simulink model "ArmModSegSep"  (R2017a)
settings: Solver=VariableStepAuto  StartTime=0.0  StopTime=length(gyroyaccel(:,1))/100  RelTol=1e-3
undefined symbols (not defined in the file): sigbuilder_block
libraries: vrlib x8, sharedtransform x6
settings Model: Creator=erich  LastModifiedBy=MarioAndres

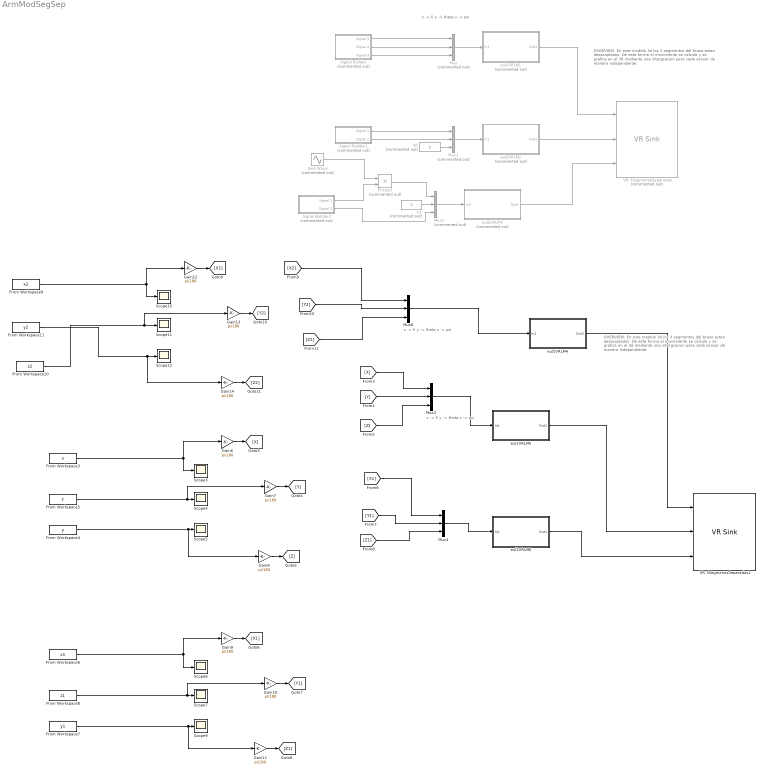
== system ArmModSegSep ==
  note: OVERVIEW:
      | En este modelo 3d los 3 segmentos del
      | brazo estan desacoplados. De esta forma
      | el movimiento se calcula y se grafica en el
      | 3d mediante una intergracion para cada
      | sensor de manera independiente.
  note: x -> fi
      | y -> theta
      | z -> psi
  note: OVERVIEW:
      | En este modelo 3d los 3 segmentos del
      | brazo estan desacoplados. De esta forma
      | el movimiento se calcula y se grafica en el
      | 3d mediante una intergracion para cada
      | sensor de manera independiente.
  note: x -> fi
      | y -> theta
      | z -> psi
  note: x -> fi
      | y -> theta
      | z -> psi
  From Workspace10 : FromWorkspace  VariableName=z2  SampleTime=0.01
  From Workspace11 : FromWorkspace  VariableName=y2  SampleTime=0.01
  From Workspace3 : FromWorkspace  VariableName=x  SampleTime=0.01
  From Workspace4 : FromWorkspace  VariableName=y  SampleTime=0.01
  From Workspace5 : FromWorkspace  VariableName=z  SampleTime=0.01
  From Workspace6 : FromWorkspace  VariableName=x1  SampleTime=0.01
  From Workspace7 : FromWorkspace  VariableName=y1  SampleTime=0.01
  From Workspace8 : FromWorkspace  VariableName=z1  SampleTime=0.01
  From Workspace9 : FromWorkspace  VariableName=x2  SampleTime=0.01
  Gain{6..14} (9 alike) : Gain  Gain=pi/180
  Mux : Mux  Commented=on  Inputs=3
  Mux1 : Mux  Commented=on  Inputs=3
  Mux2 : Mux  Commented=on  Inputs=3
  Mux3 : Mux  Inputs=3
  Mux4 : Mux  Inputs=3
  Mux6 : Mux  Inputs=3
  Product : Product  Commented=on
  Scope{3..7,9..12} (9 alike) : Scope
  Signal Builder : Subsystem  Tag=STV Subsys  Commented=on  LoadFcn=sigbuilder_block('load');  StartFcn=sigbuilder_block('start');  StopFcn=sigbuilder_block('stop');  ClipboardFcn=sigbuilder_block('clipboard');  mask(Sigbuilder block){tuvar=[0:10]}
      mask help: Simulink:masks:SigbuilderBlock_MD
      mask init:
      | if ~strcmp(get_param(bdroot(gcbh),'SimulationStatus'),'stopped') tuvar = sigbuilder_block('maskInit'); end
      settings: CopyFcn=sigbuilder_block('copy');  DeleteFcn=sigbuilder_block('delete');  ModelCloseFcn=sigbuilder_block('modelClose');  PreSaveFcn=sigbuilder_block('preSave');  PauseFcn=sigbuilder_block('pause');  ContinueFcn=sigbuilder_block('continue');  NameChangeFcn=sigbuilder_block('namechange');  OpenFcn=sigbuilder_block('open',[204 106.5 550.5 359.25 ]);  CloseFcn=sigbuilder_block('close');
      mask Display: plot(0, 0, 100, 100,[2, 2, 32, 32, 2], [68, 8, 8, 68, 68],[32, 2], [38, 38], [32, 19, 2],[53, 60, 44], [32, 17, 17, 2],[16, 16, 31, 31]);txt = getActiveGroup(gcbh);text(2, 100, txt,'verticalAlignment', 'top');
  Signal Builder1 : Subsystem  Tag=STV Subsys  Commented=on  LoadFcn=sigbuilder_block('load');  StartFcn=sigbuilder_block('start');  StopFcn=sigbuilder_block('stop');  ClipboardFcn=sigbuilder_block('clipboard');  mask(Sigbuilder block){tuvar=[0:10]}
      mask help: Simulink:masks:SigbuilderBlock_MD
      mask init:
      | if ~strcmp(get_param(bdroot(gcbh),'SimulationStatus'),'stopped') tuvar = sigbuilder_block('maskInit'); end
      settings: CopyFcn=sigbuilder_block('copy');  DeleteFcn=sigbuilder_block('delete');  ModelCloseFcn=sigbuilder_block('modelClose');  PreSaveFcn=sigbuilder_block('preSave');  PauseFcn=sigbuilder_block('pause');  ContinueFcn=sigbuilder_block('continue');  NameChangeFcn=sigbuilder_block('namechange');  OpenFcn=sigbuilder_block('open',[437.25 153 550.5 359.25 ]);  CloseFcn=sigbuilder_block('close');
      mask Display: plot(0, 0, 100, 100,[2, 2, 32, 32, 2], [68, 8, 8, 68, 68],[32, 2], [38, 38], [32, 19, 2],[53, 60, 44], [32, 17, 17, 2],[16, 16, 31, 31]);txt = getActiveGroup(gcbh);text(2, 100, txt,'verticalAlignment', 'top');
  Signal Builder2 : Subsystem  Tag=STV Subsys  Commented=on  LoadFcn=sigbuilder_block('load');  StartFcn=sigbuilder_block('start');  StopFcn=sigbuilder_block('stop');  ClipboardFcn=sigbuilder_block('clipboard');  mask(Sigbuilder block){tuvar=[0:10]}
      mask help: Simulink:masks:SigbuilderBlock_MD
      mask init:
      | if ~strcmp(get_param(bdroot(gcbh),'SimulationStatus'),'stopped') tuvar = sigbuilder_block('maskInit'); end
      settings: CopyFcn=sigbuilder_block('copy');  DeleteFcn=sigbuilder_block('delete');  ModelCloseFcn=sigbuilder_block('modelClose');  PreSaveFcn=sigbuilder_block('preSave');  PauseFcn=sigbuilder_block('pause');  ContinueFcn=sigbuilder_block('continue');  NameChangeFcn=sigbuilder_block('namechange');  OpenFcn=sigbuilder_block('open',[437.25 153 550.5 359.25 ]);  CloseFcn=sigbuilder_block('close');
      mask Display: plot(0, 0, 100, 100,[2, 2, 32, 32, 2], [68, 8, 8, 68, 68],[32, 2], [38, 38], [32, 19, 2],[53, 60, 44], [32, 17, 17, 2],[16, 16, 31, 31]);txt = getActiveGroup(gcbh);text(2, 100, txt,'verticalAlignment', 'top');
  Sine Wave : Sin  Commented=on  Amplitude=pi/10  Frequency=3  SampleTime=0
  VR 3SegmenosSeparados : vrlib/VR Sink  Commented=on  InstantiateOnLoad=on  SampleTime=0.1  ViewEnable=on  RemoteChange=off  RemoteView=off  FieldsWritten=Sphere_HombroCodo.rotation.4.1.1.double#Sphere_CodoMano.rotation.4.1.1.double#Sphere_Mano.rotation.4.1.1.double  WorldFileName=VM\VM_HCM_separados.wrl  AutoView=off  VideoDimensions=[]  AllowVariableSize=off
      settings: SourceProductBaseCode=VR
  VR 3SegmenosSeparados1 : vrlib/VR Sink  InstantiateOnLoad=on  SampleTime=0.01  ViewEnable=on  RemoteChange=off  RemoteView=off  FieldsWritten=Sphere_HombroCodo.rotation.4.1.1.double#Sphere_CodoMano.rotation.4.1.1.double#Sphere_Mano.rotation.4.1.1.double  WorldFileName=VM\VM_HCM_separados.wrl  AutoView=off  VideoDimensions=[]  AllowVariableSize=off
      settings: SourceProductBaseCode=VR
  eul2VRLM1 : Subsystem  Commented=on
  eul2VRLM2 : Subsystem  Commented=on
  eul2VRLM3 : Subsystem  Commented=on
  eul2VRLM4 : Subsystem
  eul2VRLM5 : Subsystem
  eul2VRLM6 : Subsystem
  k0 : Constant  Commented=on  Value=0
  k1 : Constant  Commented=on  Value=0
  wires:
  Signal Builder2/1(Signal 1) -> Product/2
  k1/1 -> Mux2/2
  Signal Builder2/2(Signal 2) -> Mux2/3
  Sine Wave/1 -> Product/1
  Signal Builder1/2(Signal 2) -> Mux1/2
  Product/1 -> Mux2/1
  Mux/1 -> eul2VRLM1/1(In1)
  Signal Builder1/1(Signal 1) -> Mux1/1
  Mux2/1 -> eul2VRLM3/1(In1)
  Mux1/1 -> eul2VRLM2/1(In1)
  k0/1 -> Mux1/3
  Signal Builder/2(Signal 2) -> Mux/2
  Signal Builder/3(Signal 3) -> Mux/3
  Signal Builder/1(Signal 1) -> Mux/1
  eul2VRLM1/1(Out1) -> VR 3SegmenosSeparados/1
  eul2VRLM2/1(Out1) -> VR 3SegmenosSeparados/2
  eul2VRLM3/1(Out1) -> VR 3SegmenosSeparados/3
  Mux6/1 -> eul2VRLM4/1(In1)
  From Workspace6/1 -> Gain9/1, Scope6/1
  [X2] -> Mux6/1
  Gain12/1 -> [X2]
  Gain11/1 -> [Z1]
  From Workspace8/1 -> Gain10/1, Scope7/1
  Gain14/1 -> [Z2]
  [X1] -> Mux4/1
  Gain13/1 -> [Y2]
  Gain7/1 -> [Y]
  [X] -> Mux3/1
  From Workspace9/1 -> Gain12/1, Scope10/1
  Gain10/1 -> [Y1]
  From Workspace5/1 -> Gain7/1, Scope4/1
  [Z2] -> Mux6/3
  eul2VRLM5/1(Out1) -> VR 3SegmenosSeparados1/2
  [Y1] -> Mux4/2
  [Z] -> Mux3/3
  eul2VRLM6/1(Out1) -> VR 3SegmenosSeparados1/3
  From Workspace3/1 -> Scope3/1, Gain6/1
  [Y] -> Mux3/2
  From Workspace7/1 -> Gain11/1, Scope9/1
  Gain9/1 -> [X1]
  eul2VRLM4/1(Out1) -> VR 3SegmenosSeparados1/1
  Gain6/1 -> [X]
  Gain8/1 -> [Z]
  [Y2] -> Mux6/2
  From Workspace4/1 -> Gain8/1, Scope5/1
  [Z1] -> Mux4/3
  Mux3/1 -> eul2VRLM5/1(In1)
  Mux4/1 -> eul2VRLM6/1(In1)
  From Workspace11/1 -> Gain14/1, Scope12/1
  From Workspace10/1 -> Gain13/1, Scope11/1

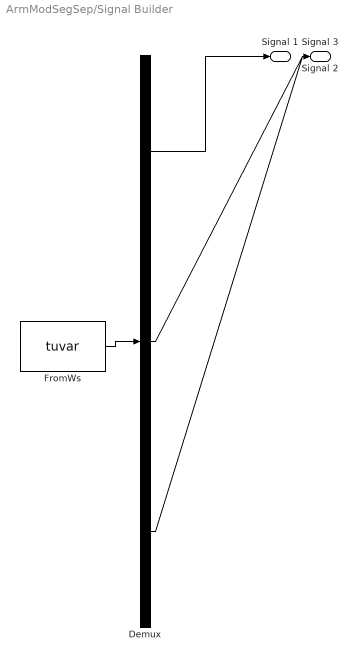
== system ArmModSegSep/Signal Builder ==
  Demux : Demux  Tag=STV Demux  Outputs=3
  FromWs : FromWorkspace  Tag=STV FromWs  VariableName=tuvar  SampleTime=0
      SigBuilderData=|
      | common.afterFinalStr = 'Extrapolate'
      | common.sampleTime = 0
      | dataSet.timeRange = [0 30]
      | dataSet.name = 'Group 1'
      | sbobj.Groups.Name = 'Group 1'
      | sbobj.Groups.Signals(1).Name = 'Signal 1'
      | sbobj.Groups.Signals(1).XData = [0 2 4 6 10 30]
      | sbobj.Groups.Signals(1).YData = [0 0 0.052 0.184 0.4 0.4]
      | sbobj.Groups.Signals(2).Name = 'Signal 2'
      | sbobj.Groups.Signals(2).XData = [0 30]
      | sbobj.Groups.Signals(2).YData = [0 0]
      | sbobj.Groups.Signals(3).Name = 'Signal 3'
      | sbobj.Groups.Signals(3).XData = [0 30]
      | sbobj.Groups.Signals(3).YData = [0 0]
      | sbobj.Groups.TimeRange = [0 30]
  Signal 1 : Outport  Tag=STV Outport
  Signal 2 : Outport  Tag=STV Outport  Port=2
  Signal 3 : Outport  Tag=STV Outport  Port=3
  wires:
  Demux/1 -> Signal 1/1
  FromWs/1 -> Demux/1
  Demux/2 -> Signal 2/1
  Demux/3 -> Signal 3/1

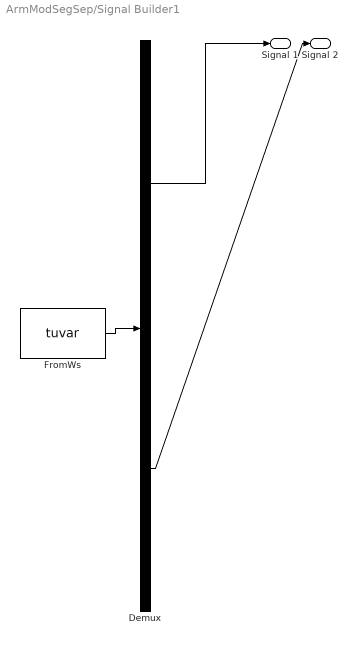
== system ArmModSegSep/Signal Builder1 ==
  Demux : Demux  Tag=STV Demux  Outputs=2
  FromWs : FromWorkspace  Tag=STV FromWs  VariableName=tuvar  SampleTime=0
      SigBuilderData=|
      | common.afterFinalStr = 'Extrapolate'
      | common.sampleTime = 0
      | dataSet.timeRange = [0 30]
      | dataSet.name = 'Group 1'
      | sbobj.Groups.Name = 'Group 1'
      | sbobj.Groups.Signals(1).Name = 'Signal 1'
      | sbobj.Groups.Signals(1).XData = [0 12 13 15 20 30]
      | sbobj.Groups.Signals(1).YData = [0 0 -0.255 -0.342 -0.308 -0.312]
      | sbobj.Groups.Signals(2).Name = 'Signal 2'
      | sbobj.Groups.Signals(2).XData = [0 30]
      | sbobj.Groups.Signals(2).YData = [0 0]
      | sbobj.Groups.TimeRange = [0 30]
  Signal 1 : Outport  Tag=STV Outport
  Signal 2 : Outport  Tag=STV Outport  Port=2
  wires:
  FromWs/1 -> Demux/1
  Demux/1 -> Signal 1/1
  Demux/2 -> Signal 2/1

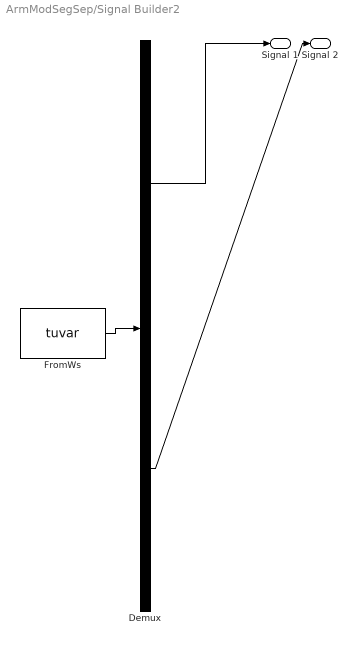
== system ArmModSegSep/Signal Builder2 ==
  Demux : Demux  Tag=STV Demux  Outputs=2
  FromWs : FromWorkspace  Tag=STV FromWs  VariableName=tuvar  SampleTime=0
      SigBuilderData=|
      | common.afterFinalStr = 'Extrapolate'
      | common.sampleTime = 0
      | dataSet.timeRange = [0 30]
      | dataSet.name = 'Group 1'
      | sbobj.Groups.Name = 'Group 1'
      | sbobj.Groups.Signals(1).Name = 'Signal 1'
      | sbobj.Groups.Signals(1).XData = [0 17 18 20 30]
      | sbobj.Groups.Signals(1).YData = [0 0 0.91 1 1]
      | sbobj.Groups.Signals(2).Name = 'Signal 2'
      | sbobj.Groups.Signals(2).XData = [0 30]
      | sbobj.Groups.Signals(2).YData = [0 0]
      | sbobj.Groups.TimeRange = [0 30]
  Signal 1 : Outport  Tag=STV Outport
  Signal 2 : Outport  Tag=STV Outport  Port=2
  wires:
  Demux/1 -> Signal 1/1
  FromWs/1 -> Demux/1
  Demux/2 -> Signal 2/1

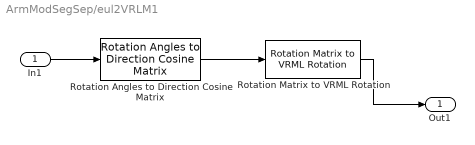
== system ArmModSegSep/eul2VRLM1 ==
  In1 : Inport
  Rotation Angles to Direction Cosine Matrix : sharedtransform/Rotation Angles to Direction Cosine Matrix  rotationOrder=ZYX
  Rotation Matrix to VRML Rotation : vrlib/Utilities/Rotation Matrix to VRML Rotation  maxzero=1e-12
      settings: SourceProductName=Simulink 3D Animation  SourceProductBaseCode=VR
  Out1 : Outport
  wires:
  Rotation Matrix to VRML Rotation/1 -> Out1/1
  In1/1 -> Rotation Angles to Direction Cosine Matrix/1
  Rotation Angles to Direction Cosine Matrix/1 -> Rotation Matrix to VRML Rotation/1

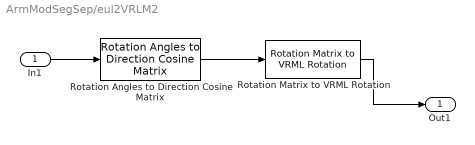
== system ArmModSegSep/eul2VRLM2 ==
  In1 : Inport
  Rotation Angles to Direction Cosine Matrix : sharedtransform/Rotation Angles to Direction Cosine Matrix  rotationOrder=ZYX
  Rotation Matrix to VRML Rotation : vrlib/Utilities/Rotation Matrix to VRML Rotation  maxzero=1e-12
      settings: SourceProductName=Simulink 3D Animation  SourceProductBaseCode=VR
  Out1 : Outport
  wires:
  Rotation Angles to Direction Cosine Matrix/1 -> Rotation Matrix to VRML Rotation/1
  In1/1 -> Rotation Angles to Direction Cosine Matrix/1
  Rotation Matrix to VRML Rotation/1 -> Out1/1

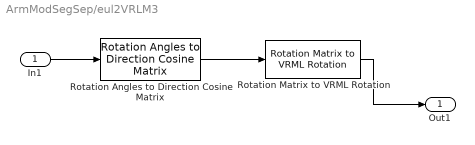
== system ArmModSegSep/eul2VRLM3 ==
  In1 : Inport
  Rotation Angles to Direction Cosine Matrix : sharedtransform/Rotation Angles to Direction Cosine Matrix  rotationOrder=ZYX
  Rotation Matrix to VRML Rotation : vrlib/Utilities/Rotation Matrix to VRML Rotation  maxzero=1e-12
      settings: SourceProductName=Simulink 3D Animation  SourceProductBaseCode=VR
  Out1 : Outport
  wires:
  Rotation Matrix to VRML Rotation/1 -> Out1/1
  In1/1 -> Rotation Angles to Direction Cosine Matrix/1
  Rotation Angles to Direction Cosine Matrix/1 -> Rotation Matrix to VRML Rotation/1

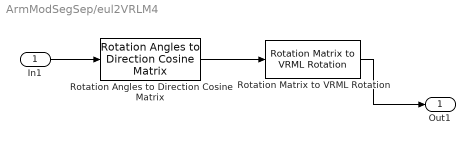
== system ArmModSegSep/eul2VRLM4 ==
  In1 : Inport
  Rotation Angles to Direction Cosine Matrix : sharedtransform/Rotation Angles to Direction Cosine Matrix  rotationOrder=ZXY
  Rotation Matrix to VRML Rotation : vrlib/Utilities/Rotation Matrix to VRML Rotation  maxzero=1e-12
      settings: SourceProductName=Simulink 3D Animation  SourceProductBaseCode=VR
  Out1 : Outport
  wires:
  Rotation Matrix to VRML Rotation/1 -> Out1/1
  In1/1 -> Rotation Angles to Direction Cosine Matrix/1
  Rotation Angles to Direction Cosine Matrix/1 -> Rotation Matrix to VRML Rotation/1

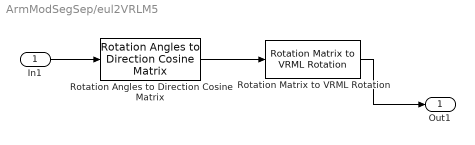
== system ArmModSegSep/eul2VRLM5 ==
  In1 : Inport
  Rotation Angles to Direction Cosine Matrix : sharedtransform/Rotation Angles to Direction Cosine Matrix  rotationOrder=ZXY
  Rotation Matrix to VRML Rotation : vrlib/Utilities/Rotation Matrix to VRML Rotation  maxzero=1e-12
      settings: SourceProductName=Simulink 3D Animation  SourceProductBaseCode=VR
  Out1 : Outport
  wires:
  Rotation Angles to Direction Cosine Matrix/1 -> Rotation Matrix to VRML Rotation/1
  In1/1 -> Rotation Angles to Direction Cosine Matrix/1
  Rotation Matrix to VRML Rotation/1 -> Out1/1

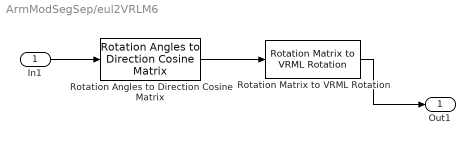
== system ArmModSegSep/eul2VRLM6 ==
  In1 : Inport
  Rotation Angles to Direction Cosine Matrix : sharedtransform/Rotation Angles to Direction Cosine Matrix  rotationOrder=ZXY
  Rotation Matrix to VRML Rotation : vrlib/Utilities/Rotation Matrix to VRML Rotation  maxzero=1e-12
      settings: SourceProductName=Simulink 3D Animation  SourceProductBaseCode=VR
  Out1 : Outport
  wires:
  Rotation Matrix to VRML Rotation/1 -> Out1/1
  In1/1 -> Rotation Angles to Direction Cosine Matrix/1
  Rotation Angles to Direction Cosine Matrix/1 -> Rotation Matrix to VRML Rotation/1
